simulink model "blockdemo"  (Simulink 6.3)
settings: Solver=FixedStepDiscrete  StartTime=0.0  StopTime=10.0  RelTol=1e-3
InitFcn:
  | %% DSPBuilder Start
  | alt_dspbuilder_update_model(bdroot)
  | %% DSPBuilder End
libraries: allblocks_alteradspbuilder2 x9
settings Model: Creator=cpurcell  LastModifiedBy=delphick
settings DebuggingCC: MultiTaskDSMMsg=error

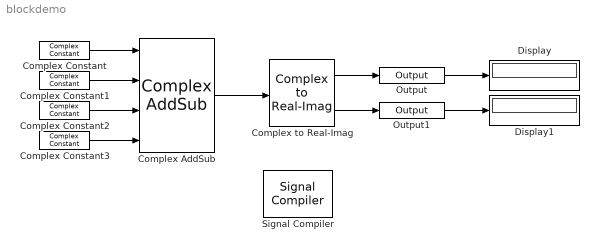
== system blockdemo ==
  Complex AddSub : allblocks_alteradspbuilder2/Complex AddSub  number_of_inputs=4  direction=+-+-  use_pipeline=on  phase_selection=1  use_ena=off  use_aclr=off
  Complex Constant : allblocks_alteradspbuilder2/Complex Constant  mask_cst_real=8  mask_cst_imag=2  BusType=Signed Integer  bwl=8  bwr=0  SpecifyClock=off
  Complex Constant1 : allblocks_alteradspbuilder2/Complex Constant  mask_cst_real=-8  mask_cst_imag=2  BusType=Signed Integer  bwl=8  bwr=0  SpecifyClock=off
  Complex Constant2 : allblocks_alteradspbuilder2/Complex Constant  mask_cst_real=8  mask_cst_imag=2  BusType=Signed Integer  bwl=8  bwr=0  SpecifyClock=off
  Complex Constant3 : allblocks_alteradspbuilder2/Complex Constant  mask_cst_real=-8  mask_cst_imag=2  BusType=Signed Integer  bwl=8  bwr=0  SpecifyClock=off
  Complex to Real-Imag : allblocks_alteradspbuilder2/Complex to Real-Imag  BusType=Signed Integer  bwl=10  bwr=0
  Display : Display
  Display1 : Display
  Output : allblocks_alteradspbuilder2/Output  iofile=C:\workspace_clean\Documentation\DesignExamples\Tutorials\UnitBlocks\Complex\ComplexAddSub\tb_blockdemo\blockdemo_Output.capture  BusType=Inferred  bwl=8  bwr=0  PORTTYPE=Output
  Output1 : allblocks_alteradspbuilder2/Output  iofile=C:\workspace_clean\Documentation\DesignExamples\Tutorials\UnitBlocks\Complex\ComplexAddSub\tb_blockdemo\blockdemo_Output1.capture  BusType=Inferred  bwl=8  bwr=0  PORTTYPE=Output
  Signal Compiler : allblocks_alteradspbuilder2/Signal Compiler  DeviceFamily=Stratix IV  DeviceName=AUTO  EnableSignalTap=off  SignalTapDepth=128  UseBoardBlock=off  StpUseDefaultClock=on  StpClock=clock
  wires:
  Complex Constant/1 -> Complex AddSub/1
  Complex Constant1/1 -> Complex AddSub/2
  Complex Constant2/1 -> Complex AddSub/3
  Complex Constant3/1 -> Complex AddSub/4
  Complex AddSub/1 -> Complex to Real-Imag/1
  Complex to Real-Imag/1 -> Output/1
  Complex to Real-Imag/2 -> Output1/1
  Output/1 -> Display/1
  Output1/1 -> Display1/1
